simulink model "a"  (R2020a)
settings: Solver=FixedStepAuto  StartTime=0.0  StopTime=10.68  FixedStep=0.01  RelTol=1e-3
undefined symbols (not defined in the file): delay, K_i
settings Model: Creator=yizha  LastModifiedBy=Brock
settings DataIOCC: ReturnWorkspaceOutputs=off
settings DebuggingCC: ArithmeticOperatorsInVariantConditions=warning
settings SFSimCC: CustomCodeUndefinedFunction=UseInterfaceOnly

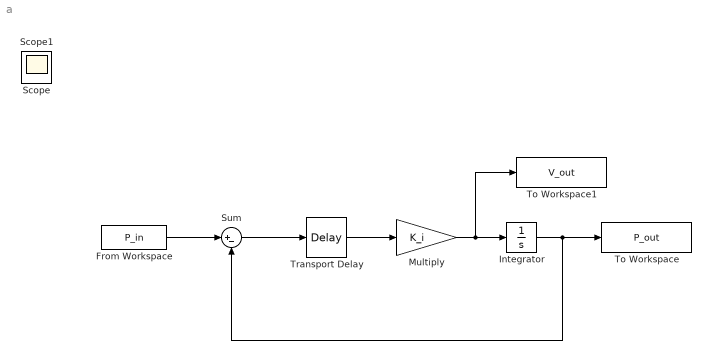
== system a ==
  From Workspace : FromWorkspace  VariableName=P_in
  Integrator : Integrator
  Multiply : Gain  Gain=K_i
  Sum : Sum  Inputs=|+-
  To Workspace : ToWorkspace  VariableName=P_out  SaveFormat=Timeseries  SampleTime=-1
  To Workspace1 : ToWorkspace  VariableName=V_out  SaveFormat=Timeseries  SampleTime=-1
  Transport Delay : TransportDelay  DelayTime=delay
  Scope : Scope
  Scope1 : Scope
  wires:
  From Workspace/1 -> Sum/1
  Sum/1 -> Transport Delay/1
  Transport Delay/1 -> Multiply/1
  Integrator/1 -> Sum/2, To Workspace/1
  Multiply/1 -> To Workspace1/1, Integrator/1
